simulink subsystem "Piero_Model"  (R2023b)
settings: Solver=VariableStepAuto  StartTime=0.0  StopTime=10.0  RelTol=1e-3
settings Model: Creator=ricfe  LastModifiedBy=ricfe

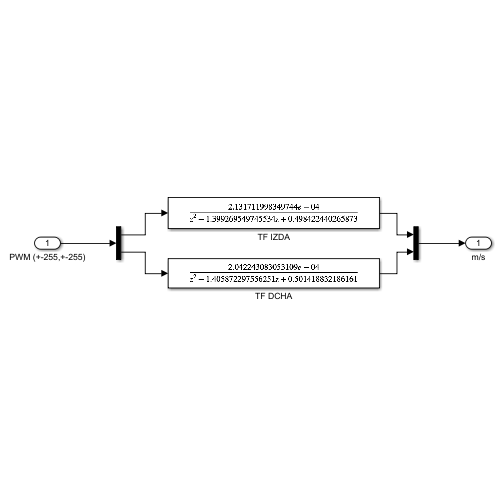
[thumbnail: Simulink's stored preview of the top-level diagram]
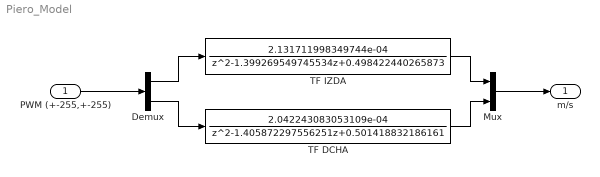
== system Piero_Model ==
  PWM (+-255,+-255) : Inport
  Demux : Demux  Outputs=2
  Mux : Mux  Inputs=2
  TF DCHA : DiscreteTransferFcn  Numerator=[2.042243083053109e-04]  Denominator=[1,-1.405872297556251,0.501418832186161]
  TF IZDA : DiscreteTransferFcn  Numerator=[2.131711998349744e-04]  Denominator=[1,-1.399269549745534,0.498422440265873]
  m/s : Outport
  wires:
  PWM (+-255,+-255)/1 -> Demux/1
  Demux/1 -> TF IZDA/1
  TF IZDA/1 -> Mux/1
  Demux/2 -> TF DCHA/1
  TF DCHA/1 -> Mux/2
  Mux/1 -> m/s/1
